simulink model "Advanced_trial"  (R2025b)
settings: Solver=VariableStepAuto  StartTime=0.0  StopTime=30  RelTol=1e-3
model workspace (MAT data in the model file):
  b = Simulink.Parameter
  b.Value = [0.5; 0.4; 0.25; 0.2; 2; 1.5; 0.02; 0.01; 9.81; 50; 50; 10; 10]
  b.Complexity = 'real'
  b.Dimensions = [13 1]
  b.DataType = 'auto'
values from neighbouring files (symbols this model uses):
  motor = [b1; b2; d1; d2]    [init_params.m]
  params = [ ... (first row only)    [init_params.m]
settings Model: Creator=DELL  LastModifiedBy=DELL

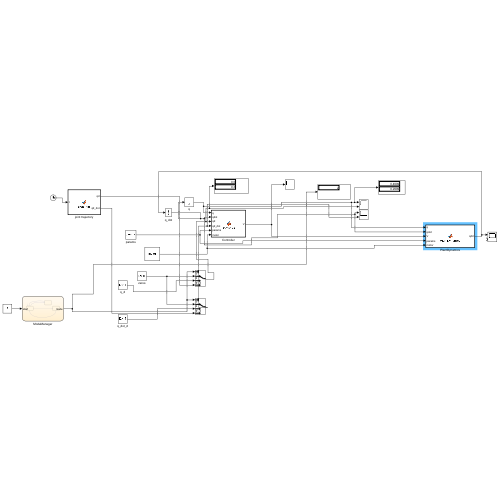
[thumbnail: Simulink's stored preview of the top-level diagram]
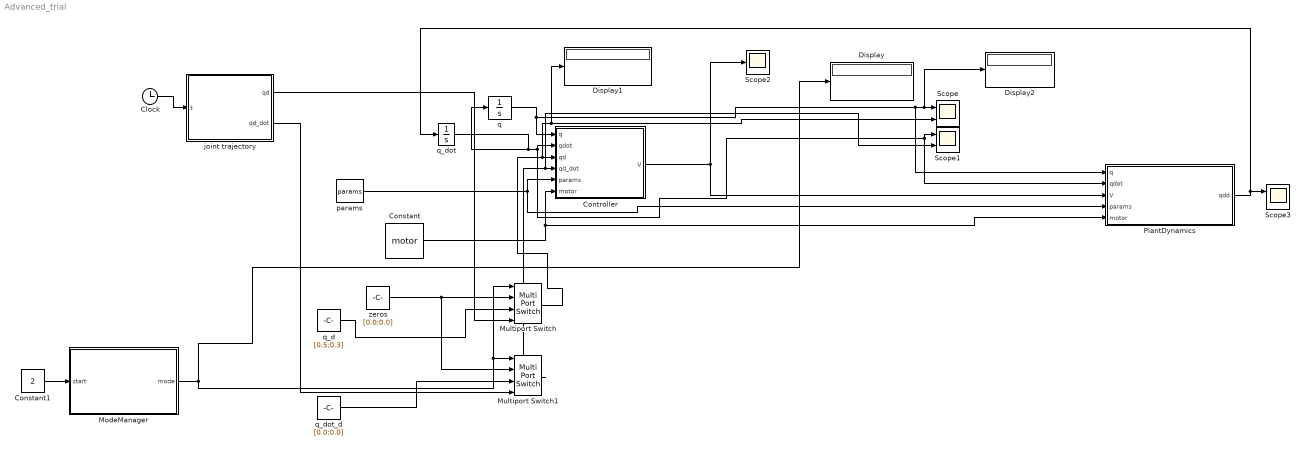
== system Advanced_trial ==
  Clock : Clock
  Constant : Constant  Value=motor
  Constant1 : Constant  Value=2
  Controller : MATLAB Function  TreatAsAtomicUnit=on
  Display : Display
  Display1 : Display
  Display2 : Display
  ModeManager : Stateflow chart  TreatAsAtomicUnit=on
  Multiport Switch : MultiPortSwitch  SaturateOnIntegerOverflow=off  InputSameDT=off
  Multiport Switch1 : MultiPortSwitch  SaturateOnIntegerOverflow=off  InputSameDT=off
  PlantDynamics : MATLAB Function  TreatAsAtomicUnit=on
  Scope : Scope  NumInputPorts=2
      settings: ActiveDisplayYMinimum=-0.065204134845508507  ActiveDisplayYMaximum=0.58683721360957675
  Scope1 : Scope  NumInputPorts=2
      settings: ActiveDisplayYMinimum=-0.27680835225219091  ActiveDisplayYMaximum=0.98324983718438141
  Scope2 : Scope
      settings: ActiveDisplayYMinimum=-0.028740255899114248  ActiveDisplayYMaximum=0.27563900855665158  DataLoggingVariableName=ScopeData2
  Scope3 : Scope  NumInputPorts=2
      settings: ActiveDisplayYMinimum=-1  ActiveDisplayYMaximum=1  DataLoggingVariableName=ScopeData3
  joint trajectory : MATLAB Function  TreatAsAtomicUnit=on
  params : Constant  Value=params
  q : Integrator  InitialCondition=[0; 0]
  q_d : Constant  Value=[0.5;0.3]
  q_dot : Integrator
  q_dot_d : Constant  Value=[0.0;0.0]
  zeros : Constant  Value=[0.0;0.0]
  wires:
  q/1 -> Controller/1(q), PlantDynamics/1(q), Display2/1, Scope/1
  q_dot/1 -> q/1, PlantDynamics/2(qdot), Scope1/1, Controller/2(qdot)
  params/1 -> Controller/5(params), PlantDynamics/4(params)
  PlantDynamics/1(qdd) -> q_dot/1, Scope3/1
  Constant/1 -> PlantDynamics/5(motor), Controller/6(motor)
  Constant1/1 -> ModeManager/1(start)
  ModeManager/1(mode) -> Display/1, Multiport Switch1/1, Multiport Switch/1
  Clock/1 -> joint trajectory/1(t)
  zeros/1 -> Multiport Switch1/2, Multiport Switch/2
  Controller/1(V) -> Scope2/1, PlantDynamics/3(V)
  q_dot_d/1 -> Multiport Switch1/3
  q_d/1 -> Multiport Switch/3
  Multiport Switch/1 -> Scope/2, Display1/1, Controller/3(qd)
  joint trajectory/1(qd) -> Multiport Switch/4
  joint trajectory/2(qd_dot) -> Multiport Switch1/4
  Multiport Switch1/1 -> Scope1/2, Controller/4(qd_dot)

== matlab function Advanced_trial/joint trajectory ==
  data: t input; qd output; qd_dot output
function [qd, qd_dot] = circle_traj(t)
R = 0.3;          % circle radius
w = 0.5;          % angular speed

qd1 = R * cos(w*t);
qd2 = R * sin(w*t);

qd = [qd1; qd2];

qd_dot = [-R*w*sin(w*t);
           R*w*cos(w*t)];
end

== matlab function Advanced_trial/Controller ==
  data: q input size=[2 1]; V output size=[2 1]; qdot input size=[2 1]; qd input size=[2 1]; qd_dot input size=[2 1]; params input size=[17 1]; motor input
function V = Controller(q, qdot, qd, qd_dot, params, motor)
% Controller outputs motor voltage V (2x1)
% All physical totals (masses/inertias) already computed in init_params.m

% --- unpack params
l1 = params(1);
l2 = params(2);
a1 = params(3);
a2 = params(4);

m1_total = params(5);   % total link1 mass
m2_total = params(6);   % total link2 mass

I1_total = params(7);   % total inertia at joint1
I2_total = params(8);   % total inertia at joint2

g = params(9);

kp1 = params(10); kp2 = params(11);
kd1 = params(12); kd2 = params(13);

Kp = diag([kp1 kp2]);
Kd = diag([kd1 kd2]);

% --- motor electrical params
b1 = motor(1); b2 = motor(2);
d1 = motor(3); d2 = motor(4);

B = diag([b1 b2]);
D = diag([d1 d2]);

% --- unpack states
q1 = q(1); q2 = q(2);
dq1 = qdot(1); dq2 = qdot(2);

% --- inertia matrix M(q)
c2 = cos(q2);

M11 = I1_total + I2_total + ...
       m1_total*a1^2 + ...
       m2_total*(l1^2 + a2^2 + 2*l1*a2*c2);

M12 = I2_total + m2_total*(a2^2 + l1*a2*c2);
M22 = I2_total + m2_total*a2^2;

M = [M11 M12; M12 M22];

% --- Coriolis term
h = - m2_total*l1*a2*sin(q2);
Cqdot = [
    h*(2*dq1 + dq2)*dq2;
    h*(dq1^2)
];

% --- gravity term
G1 = m1_total*a1*g*cos(q1) + ...
     m2_total*g*(l1*cos(q1) + a2*cos(q1+q2));

G2 = m2_total*a2*g*cos(q1+q2);
G = [G1; G2];

% --- PD tracking control
qd_ddot = [0; 0];    % zero acceleration for regulation

e = qd - q;
edot = qd_dot - qdot;

v = qd_ddot + Kd*edot + Kp*e;

% --- desired torque
tau_des = M*v + Cqdot + G;

% --- voltage:  V = B^{-1} (tau_des + D*qdot)
V = B \ (tau_des + D*qdot);

end

== stateflow chart Advanced_trial/ModeManager ==
  state POS
    entry:
    mode=2;
  state OFF
    entry:
    mode=1;
  state CIRCLE
    entry:
    mode=3;
  POS -> OFF : [start==0
      | ]
  OFF -> POS [order 2] : [start==2]
  (default) -> OFF
  OFF -> CIRCLE [order 1] : [start==1]
  CIRCLE -> OFF : [start == 0]
  data: start input; mode output

== matlab function Advanced_trial/PlantDynamics ==
  data: q input; qdd output; qdot input; V input; params input; motor input
function qdd = PlantDynamics(q, qdot, V, params, motor)
% Electromechanical plant using PRECOMPUTED total inertias & masses
% All PAT and motor effects already handled inside init_params.m

% --- unpack params (precomputed totals)
l1 = params(1); 
l2 = params(2);
a1 = params(3);
a2 = params(4);

m1_total = params(5);   % total mass link1 + motor1
m2_total = params(6);   % total mass link2 + motor2

I1_total = params(7);   % joint1 total inertia
I2_total = params(8);   % joint2 total inertia

g = params(9);

% --- motor electrical params
b1 = motor(1); b2 = motor(2);
d1 = motor(3); d2 = motor(4);

B = diag([b1 b2]);
D = diag([d1 d2]);

% --- states
q1 = q(1);   q2 = q(2);
dq1 = qdot(1); dq2 = qdot(2);

% --- inertia matrix M(q)
c2 = cos(q2);

M11 = I1_total + I2_total + ...
       m1_total*a1^2 + ...
       m2_total*(l1^2 + a2^2 + 2*l1*a2*c2);

M12 = I2_total + m2_total*(a2^2 + l1*a2*c2);
M22 = I2_total + m2_total*a2^2;

M = [M11  M12;
     M12  M22];

% --- Coriolis/Centrifugal C(q,qdot)*qdot
h = - m2_total*l1*a2*sin(q2);
Cqdot = [
    h*(2*dq1 + dq2)*dq2;
    h*(dq1^2)
];

% --- gravity torques
G1 = m1_total*a1*g*cos(q1) + ...
     m2_total*g*(l1*cos(q1) + a2*cos(q1+q2));

G2 = m2_total*a2*g*cos(q1+q2);
G = [G1; G2];

% --- motor torque: tau = B*V - D*qdot
tau = B*V - D*qdot;

% --- acceleration
qdd = M \ (tau - Cqdot - G);
end
